simulink model "InvPendOutputFeedback_PolePlacement"  (R2023b)
settings: Solver=VariableStepAuto  StartTime=0.0  StopTime=10  RelTol=1e-3
values from neighbouring files (symbols this model uses):
  A = [0      1              0           0 ... (first row only)    [InvPendModel.m]
  Aobs = A-L*C    [InvPendModel.m]
  B = [     0 ... (first row only)    [InvPendModel.m]
  Bobs = [L B-L*D]    [InvPendModel.m]
  C = [1 0 0 0 ... (first row only)    [InvPendModel.m]
  Cobs = eye(4)    [InvPendModel.m]
  D = [0 ... (first row only)    [InvPendModel.m]
  Dobs = zeros(4,3)    [InvPendModel.m]
  Kf = K(:,1:4)    [InvPendModel.m]
  Ki = K(:,end)    [InvPendModel.m]
settings Model: Creator=alfredo  LastModifiedBy=roberto_ambrosino
settings SolverCC: AlgebraicLoopSolver=TrustRegion
settings DataIOCC: ReturnWorkspaceOutputs=off
settings DebuggingCC: UnconnectedInputMsg=warning  UnconnectedOutputMsg=warning  UnconnectedLineMsg=warning  ArithmeticOperatorsInVariantConditions=warning
settings ModelReferenceCC: EnableRefExpFcnMdlSchedulingChecks=on
settings SFSimCC: SimUseLocalCustomCode=off  CustomCodeUndefinedFunction=UseInterfaceOnly
settings RTWCC: RTWUseLocalCustomCode=off

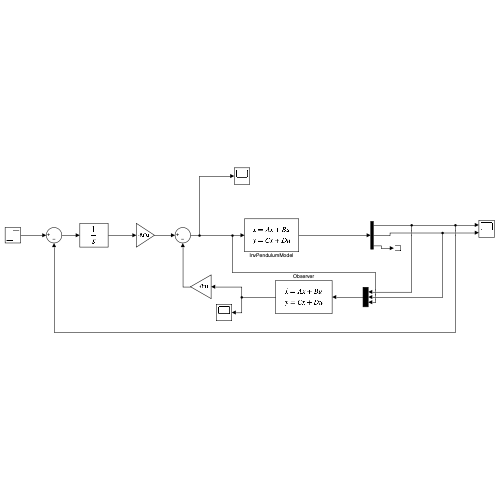
[thumbnail: Simulink's stored preview of the top-level diagram]
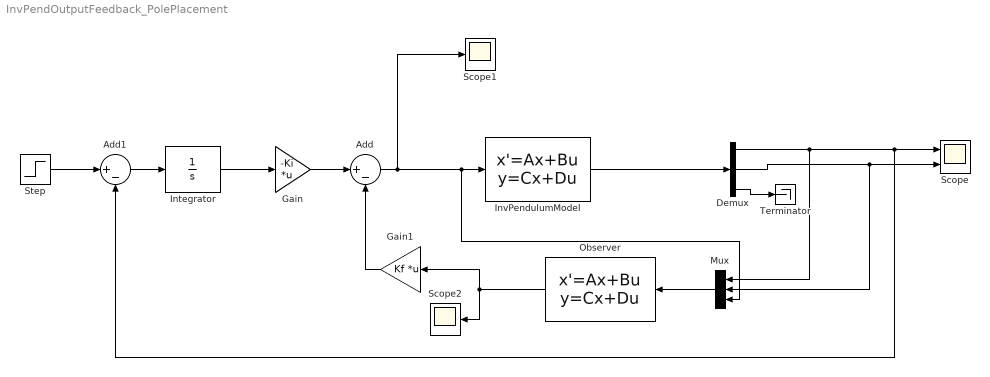
== system InvPendOutputFeedback_PolePlacement ==
  Add : Sum  Inputs=|+-
  Add1 : Sum  Inputs=|+-
  Demux : Demux  Outputs=[1 1 4]
  Gain : Gain  Gain=-Ki  Multiplication=Matrix(K*u)
  Gain1 : Gain  Gain=Kf  Multiplication=Matrix(K*u)
  Integrator : Integrator
  InvPendulumModel : StateSpace  A=A  B=B  C=[C;eye(4)]  D=[D;zeros(4,1)]  InitialCondition=[0;0;0.1;.0]
  Mux : Mux  Inputs=3
  Observer : StateSpace  A=Aobs  B=Bobs  C=Cobs  D=Dobs  InitialCondition=0
  Scope : Scope  NumInputPorts=2
  Scope1 : Scope
  Scope2 : Scope
  Step : Step  Time=0.1  SampleTime=0
  Terminator : Terminator
  wires:
  Integrator/1 -> Gain/1
  Add/1 -> Scope1/1, Mux/3, InvPendulumModel/1
  Gain/1 -> Add/1
  InvPendulumModel/1 -> Demux/1
  Gain1/1 -> Add/2
  Add1/1 -> Integrator/1
  Step/1 -> Add1/1
  Demux/1 -> Mux/1, Add1/2, Scope/1
  Demux/2 -> Mux/2, Scope/2
  Mux/1 -> Observer/1
  Observer/1 -> Scope2/1, Gain1/1
  Demux/3 -> Terminator/1
